simulink model "FS"  (R2020a)
settings: Solver=VariableStepAuto  StartTime=0.0  StopTime=10.0  RelTol=1e-3
values from neighbouring files (symbols this model uses):
  g = 9.807    [variables.m]
  Jb = 0.001304    [variables.m]
  Jw = 0.0000241    (= 2.41e-05)    [variables.m]
  l = 0.04    [variables.m]
  mb = 0.660    (= 0.66)    [variables.m]
  mwa = 0.104    [variables.m]
  R = 0.031    [variables.m]
settings Model: Creator=Acer  LastModifiedBy=Acer

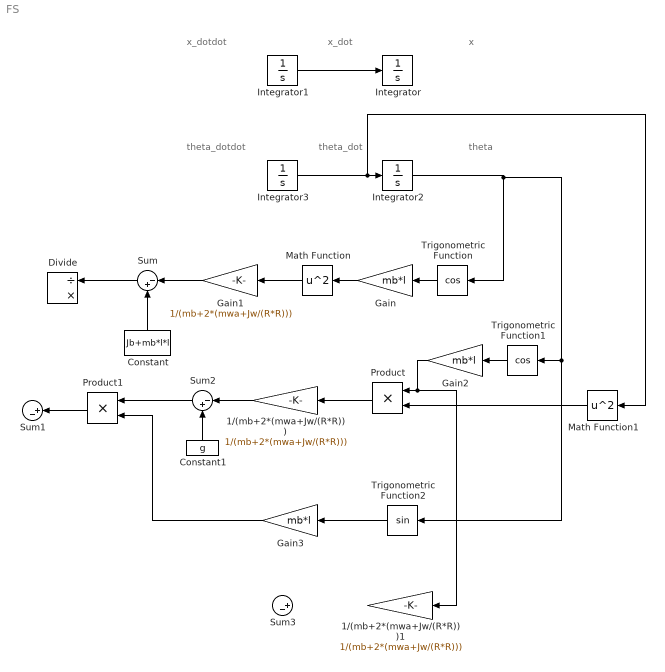
== system FS ==
  note: x_dot
  note: x_dotdot
  note: x
  note: theta
  note: theta_dotdot
  note: theta_dot
  1/(mb+2*(mwa+Jw/(R*R))) : Gain  Gain=1/(mb+2*(mwa+Jw/(R*R)))
  1/(mb+2*(mwa+Jw/(R*R)))1 : Gain  Gain=1/(mb+2*(mwa+Jw/(R*R)))
  Constant : Constant  Value=Jb+mb*l*l
  Constant1 : Constant  Value=g
  Divide : Product  Inputs=/*
  Gain : Gain  Gain=mb*l
  Gain1 : Gain  Gain=1/(mb+2*(mwa+Jw/(R*R)))
  Gain2 : Gain  Gain=mb*l
  Gain3 : Gain  Gain=mb*l
  Integrator{,1..3} (4 alike) : Integrator
  Math Function : Math  Operator=square  SaturateOnIntegerOverflow=on
  Math Function1 : Math  Operator=square  SaturateOnIntegerOverflow=on
  Product : Product
  Product1 : Product
  Sum : Sum  Inputs=|-+
  Sum1 : Sum  Inputs=|+-
  Sum2 : Sum  Inputs=|-+
  Sum3 : Sum  Inputs=|+-
  Trigonometric Function : Trigonometry  Operator=cos
  Trigonometric Function1 : Trigonometry  Operator=cos
  Trigonometric Function2 : Trigonometry
  wires:
  Integrator1/1 -> Integrator/1
  Integrator3/1 -> Math Function1/1, Integrator2/1
  Integrator2/1 -> Trigonometric Function2/1, Trigonometric Function1/1, Trigonometric Function/1
  Trigonometric Function/1 -> Gain/1
  Gain/1 -> Math Function/1
  Math Function/1 -> Gain1/1
  Gain1/1 -> Sum/1
  Constant/1 -> Sum/2
  Sum/1 -> Divide/1
  Trigonometric Function1/1 -> Gain2/1
  Gain2/1 -> 1/(mb+2*(mwa+Jw/(R*R)))1/1, Product/1
  Math Function1/1 -> Product/2
  Product/1 -> 1/(mb+2*(mwa+Jw/(R*R)))/1
  1/(mb+2*(mwa+Jw/(R*R)))/1 -> Sum2/1
  Constant1/1 -> Sum2/2
  Trigonometric Function2/1 -> Gain3/1
  Sum2/1 -> Product1/1
  Gain3/1 -> Product1/2
  Product1/1 -> Sum1/1
